simulink library "rocofLS"  (Simulink 8.5)
settings: Solver=ode5  SolverMode=SingleTasking  StartTime=0.0  StopTime=Inf  FixedStep=0.001  RelTol=1e-3
libraries: commfilt2 x7, powerlib_meascontrol x2
settings Model: Creator=Administrator  LastModifiedBy=Administrator

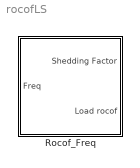
== system rocofLS ==
  Rocof_Freq : Subsystem  TreatAsAtomicUnit=on  SystemSampleTime=20e-3  mask{DT=0.8}
      mask prompts: DT "RocofFreqdelay time (s):"
      mask init:
      | Delay=DT;

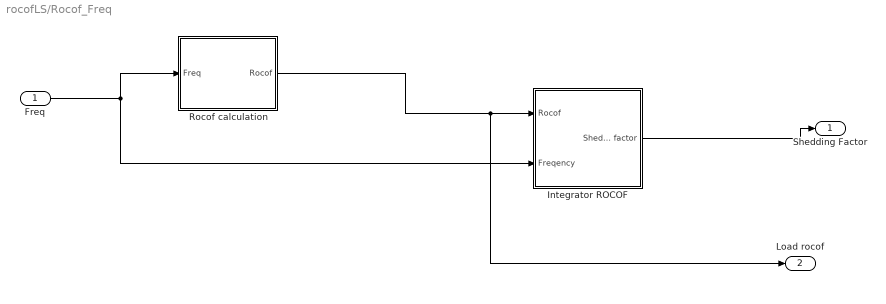
== system rocofLS/Rocof_Freq ==
  Freq : Inport
  Integrator ROCOF : Subsystem
  Rocof calculation : Subsystem  SystemSampleTime=20e-3
  Shedding Factor : Outport
  Load rocof : Outport  Port=2
  wires:
  Rocof calculation/1(Rocof) -> Load rocof/1, Integrator ROCOF/1(Rocof)
  Integrator ROCOF/1(Shedding factor) -> Shedding Factor/1
  Freq/1 -> Rocof calculation/1(Freq), Integrator ROCOF/2(Freqency)

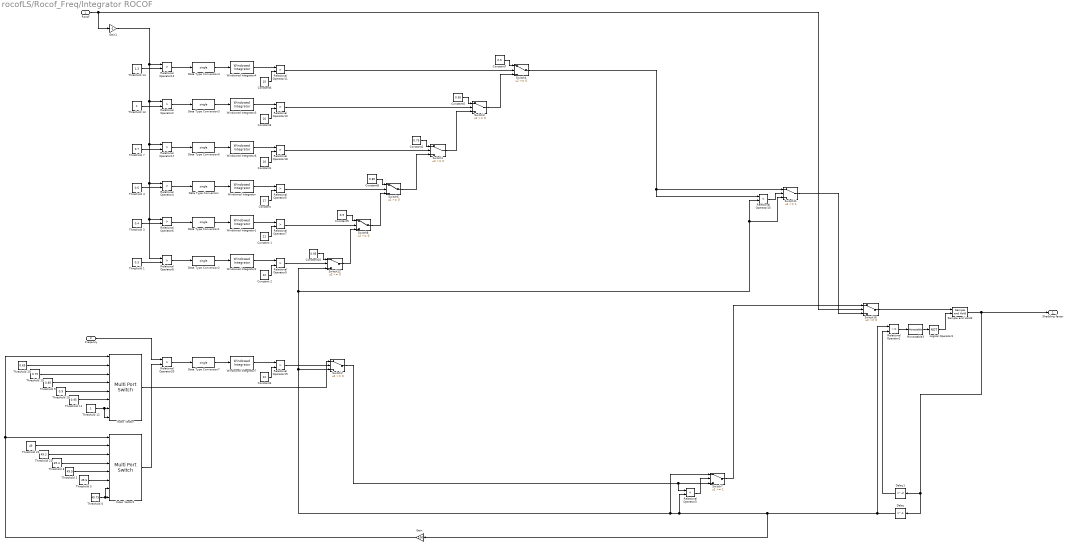
== system rocofLS/Rocof_Freq/Integrator ROCOF ==
  Rocof : Inport
  Freqency : Inport  Port=2
  Constant : Constant  Value=17
  Constant 1 : Constant  Value=21
  Constant 2 : Constant  Value=22
  Constant1 : Constant  Value=16
  Constant10 : Constant  Value=0.95
  Constant2 : Constant  Value=0.75
  Constant3 : Constant  Value=16
  Constant4 : Constant  Value=22
  Constant5 : Constant  Value=0.65
  Constant6 : Constant  Value=15
  Constant7 : Constant  Value=0.5
  Constant8 : Constant  Value=0.85
  Constant9 : Constant  Value=0.9
  Data Type Conversion{,1..4,6..7} (7 alike) : DataTypeConversion  OutDataTypeStr=single
  Delay : Delay  DelayLength=1  InitialCondition=1
  Delay1 : Delay  InitialCondition=1
  Gain : Gain  Gain=100
  Gain1 : Gain  Gain=-1
  Index Vector : MultiPortSwitch  DataPortOrder=Specify indices  Inputs=4  DataPortIndices={50,65,75,85,90,95,100}
  Index Vector1 : MultiPortSwitch  DataPortOrder=Specify indices  Inputs=4  DataPortIndices={50,65,75,85,90,95,100}
  Logical Operator3 : Logic  Operator=NOT  AllPortsSameDT=off  OutDataTypeStr=boolean
  Monostable3 : powerlib_meascontrol/Logic/Monostable  EdgeDetect=Rising  PulseDuration=4  ic=0  Ts=20e-3
  Relational Operator1 : RelationalOperator  Operator=~=  OutDataTypeStr=boolean
  Relational Operator{2,4..12,17..20} (14 alike) : RelationalOperator  Operator=>  OutDataTypeStr=boolean
  Relational Operator15 : RelationalOperator  Operator=<  OutDataTypeStr=boolean
  Relational Operator3 : RelationalOperator  Operator=<  OutDataTypeStr=boolean
  Sample and Hold3 : powerlib_meascontrol/Additional Components/Sample and Hold  ic=1  Ts=20e-3
  Switch{1..4,6,8,12,16} (8 alike) : Switch
  Switch11 : Switch  Threshold=1
  Switch7 : Switch  Threshold=1
  Threshold 1 : Constant  Value=0.3
  Threshold 10 : Constant  Value=0.9
  Threshold 11 : Constant  Value=0.95
  Threshold 12 : Constant
  Threshold 13 : Constant
  Threshold 14 : Constant  Value=1.3
  Threshold 19 : Constant  Value=0.75
  Threshold 2 : Constant  Value=49.5
  Threshold 20 : Constant  Value=0.65
  Threshold 21 : Constant  Value=49.2
  Threshold 22 : Constant  Value=49
  Threshold 3 : Constant  Value=0.4
  Threshold 4 : Constant  Value=0.6
  Threshold 5 : Constant  Value=49.6
  Threshold 6 : Constant  Value=49.75
  Threshold 7 : Constant  Value=0.7
  Threshold 8 : Constant  Value=49.4
  Threshold 9 : Constant  Value=0.85
  Windowed Integrator{,1..4,6..7} (7 alike) : commfilt2/Windowed Integrator  integperiod=25  roundingMode=Floor  overflowMode=off  InputProcessing=Columns as channels (frame based)
  Shedding factor : Outport
  wires:
  Threshold 4/1 -> Relational Operator4/2
  Relational Operator5/1 -> Switch6/2
  Relational Operator4/1 -> Data Type Conversion/1
  Windowed Integrator1/1 -> Relational Operator7/1
  Constant 1/1 -> Relational Operator7/2
  Relational Operator7/1 -> Switch8/2
  Windowed Integrator2/1 -> Relational Operator9/1
  Relational Operator9/1 -> Switch12/2
  Windowed Integrator/1 -> Relational Operator5/1
  Constant/1 -> Relational Operator5/2
  Constant 2/1 -> Relational Operator9/2
  Threshold 3/1 -> Relational Operator6/2
  Relational Operator6/1 -> Data Type Conversion1/1
  Constant9/1 -> Switch8/1
  Constant8/1 -> Switch6/1
  Gain1/1 -> Relational Operator12/1, Relational Operator2/1, Relational Operator17/1, Relational Operator4/1, Relational Operator8/1, Relational Operator6/1
  Relational Operator8/1 -> Data Type Conversion2/1
  Threshold 1/1 -> Relational Operator8/2
  Constant10/1 -> Switch12/1
  Switch12/1 -> Switch8/3
  Switch8/1 -> Switch6/3
  Freqency/1 -> Relational Operator20/1
  Data Type Conversion/1 -> Windowed Integrator/1
  Data Type Conversion1/1 -> Windowed Integrator1/1
  Data Type Conversion2/1 -> Windowed Integrator2/1
  Switch2/1 -> Relational Operator3/1, Switch7/3
  Relational Operator3/1 -> Switch7/2
  Rocof/1 -> Switch16/2, Gain1/1
  Relational Operator15/1 -> Switch11/2
  Delay1/1 -> Relational Operator1/2
  Switch11/1 -> Switch16/3
  Logical Operator3/1 -> Sample and Hold3/2
  Monostable3/1 -> Logical Operator3/1
  Relational Operator1/1 -> Monostable3/1
  Switch16/1 -> Sample and Hold3/1
  Switch7/1 -> Switch16/1
  Sample and Hold3/1 -> Shedding factor/1, Delay/1, Delay1/1
  Threshold 7/1 -> Relational Operator17/2
  Relational Operator18/1 -> Switch1/2
  Relational Operator17/1 -> Data Type Conversion6/1
  Windowed Integrator6/1 -> Relational Operator18/1
  Constant1/1 -> Relational Operator18/2
  Constant2/1 -> Switch1/1
  Data Type Conversion6/1 -> Windowed Integrator6/1
  Switch6/1 -> Switch1/3
  Switch1/1 -> Switch3/3
  Constant4/1 -> Relational Operator19/2
  Index Vector1/1 -> Relational Operator20/2
  Relational Operator20/1 -> Data Type Conversion7/1
  Windowed Integrator7/1 -> Relational Operator19/1
  Data Type Conversion7/1 -> Windowed Integrator7/1
  Relational Operator19/1 -> Switch2/2
  Index Vector/1 -> Switch2/1
  Delay/1 -> Switch2/3, Switch12/3, Switch11/3, Relational Operator15/2, Switch7/1, Relational Operator3/2, Gain/1, Relational Operator1/1
  Gain/1 -> Index Vector1/1, Index Vector/1
  Threshold 13/1 -> Relational Operator2/2
  Relational Operator10/1 -> Switch3/2
  Relational Operator2/1 -> Data Type Conversion3/1
  Windowed Integrator3/1 -> Relational Operator10/1
  Constant3/1 -> Relational Operator10/2
  Constant5/1 -> Switch3/1
  Data Type Conversion3/1 -> Windowed Integrator3/1
  Threshold 14/1 -> Relational Operator12/2
  Relational Operator11/1 -> Switch4/2
  Relational Operator12/1 -> Data Type Conversion4/1
  Windowed Integrator4/1 -> Relational Operator11/1
  Constant6/1 -> Relational Operator11/2
  Constant7/1 -> Switch4/1
  Data Type Conversion4/1 -> Windowed Integrator4/1
  Switch3/1 -> Switch4/3
  Switch4/1 -> Relational Operator15/1, Switch11/1
  Threshold 12/1 -> Index Vector/8, Index Vector/7
  Threshold 11/1 -> Index Vector/6
  Threshold 10/1 -> Index Vector/5
  Threshold 9/1 -> Index Vector/4
  Threshold 19/1 -> Index Vector/3
  Threshold 20/1 -> Index Vector/2
  Threshold 6/1 -> Index Vector1/8, Index Vector1/7
  Threshold 5/1 -> Index Vector1/6
  Threshold 2/1 -> Index Vector1/5
  Threshold 8/1 -> Index Vector1/4
  Threshold 21/1 -> Index Vector1/3
  Threshold 22/1 -> Index Vector1/2

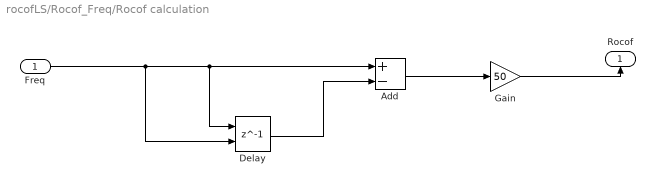
== system rocofLS/Rocof_Freq/Rocof calculation ==
  Freq : Inport
  Add : Sum  Inputs=+-
  Delay : Delay  DelayLength=1  InitialConditionSource=Input port
      settings: InputPortMap=u0,p4
  Gain : Gain  Gain=50
  Rocof : Outport
  wires:
  Gain/1 -> Rocof/1
  Freq/1 -> Delay/2, Delay/1, Add/1
  Delay/1 -> Add/2
  Add/1 -> Gain/1
